simulink model "FanSpd_DD"  (R2016b)
settings: configuration reference "CodeGenConfigSet" (kept outside this file)
values from neighbouring files (symbols this model uses):
  Fan_bSwtPrs_C = Calibration.Parameter    [init_FanSpd_DD.m]    (also in init_FanSpd_DD_SIL.m = Simulink.Parameter)
  Fan_numImpRev_C = Calibration.Parameter    [init_FanSpd_DD.m]    (also in init_FanSpd_DD_SIL.m = Simulink.Parameter)
settings Model: Creator=xinchangran  LastModifiedBy=xinchangran
settings ConfigSetRef: SourceLocation=Base Workspace

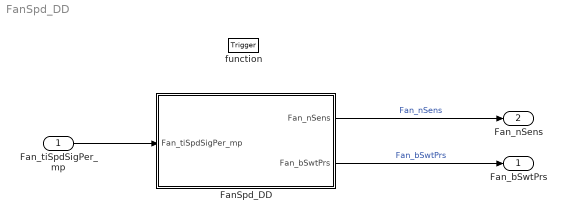
== system FanSpd_DD ==
  Fan_tiSpdSigPer_mp : Inport  Tag=us  Description=Time between two pulses of fan speed sensor  OutMin=0  OutMax=6553  OutDataTypeStr=Period_us
  function : TriggerPort  TriggerType=function-call  VariantControl=Variant
  FanSpd_DD : Subsystem
  Fan_bSwtPrs : Outport  Description=Fan_bSwtPrs ==0 fan sensor is not installed/==1 sensor stalled  OutMin=0  OutMax=1  OutDataTypeStr=boolean
  Fan_nSens : Outport  Tag=rpm  Description=Sensed fan speed  Port=2  OutMin=0  OutMax=32767  OutDataTypeStr=FanSpd_rpm
  wires:
  Fan_tiSpdSigPer_mp/1 -> FanSpd_DD/1(Fan_tiSpdSigPer_mp)
  FanSpd_DD/1(Fan_nSens) -> Fan_nSens/1  "Fan_nSens"
  FanSpd_DD/2(Fan_bSwtPrs) -> Fan_bSwtPrs/1  "Fan_bSwtPrs"

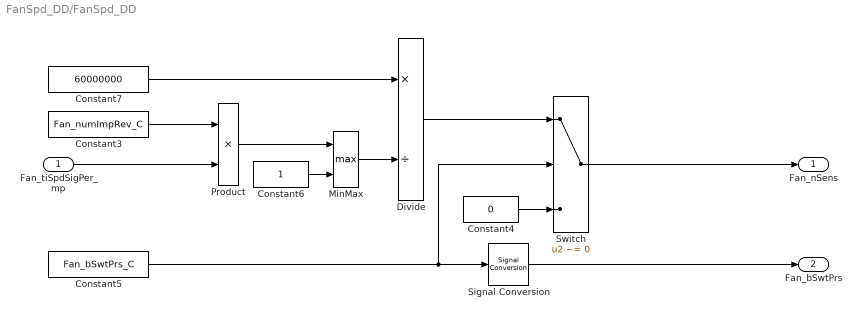
== system FanSpd_DD/FanSpd_DD ==
  Fan_tiSpdSigPer_mp : Inport  Tag=us  OutMin=0  OutMax=6553  OutDataTypeStr=Period_us
  Constant3 : Constant  Value=Fan_numImpRev_C
  Constant4 : Constant  Value=0  OutDataTypeStr=Inherit: Inherit via back propagation
  Constant5 : Constant  Value=Fan_bSwtPrs_C  OutMin=0  OutMax=1  SampleTime=-1
  Constant6 : Constant  OutDataTypeStr=Inherit: Inherit via back propagation
  Constant7 : Constant  Value=60000000  OutDataTypeStr=Counter_num  LockScale=on
  Divide : Product  Inputs=*/  OutDataTypeStr=Inherit: Inherit via back propagation  SaturateOnIntegerOverflow=on
  MinMax : MinMax  Function=max  Inputs=2  OutDataTypeStr=Inherit: Inherit via back propagation
  Product : Product  OutDataTypeStr=Inherit: Inherit via back propagation  SaturateOnIntegerOverflow=on
  Signal Conversion : SignalConversion  OverrideOpt=on
  Switch : Switch  Criteria=u2 ~= 0  SaturateOnIntegerOverflow=on  InputSameDT=on
  Fan_nSens : Outport  Tag=rpm  OutMin=0  OutMax=32767  OutDataTypeStr=FanSpd_rpm
  Fan_bSwtPrs : Outport  Port=2
  wires:
  Constant3/1 -> Product/1
  Divide/1 -> Switch/1
  Constant4/1 -> Switch/3
  MinMax/1 -> Divide/2
  Product/1 -> MinMax/1
  Switch/1 -> Fan_nSens/1
  Fan_tiSpdSigPer_mp/1 -> Product/2
  Constant6/1 -> MinMax/2
  Signal Conversion/1 -> Fan_bSwtPrs/1
  Constant7/1 -> Divide/1
  Constant5/1 -> Switch/2, Signal Conversion/1
